simulink model "DroneSim"  (R2026a)
settings: Solver=ode45  StopTime=20
undefined symbols (not defined in the file): A, B, Cobs, Klqr, Kr, Lobs, pVec, T_eq, u_eq, windStr, x0
libraries: simulink x3, cstblocks_varying x3
settings Model: Creator=bryon  LastModifiedBy=bryon

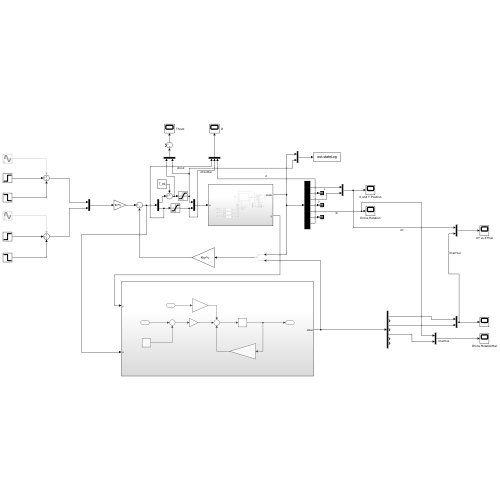
[thumbnail: Simulink's stored preview of the top-level diagram]
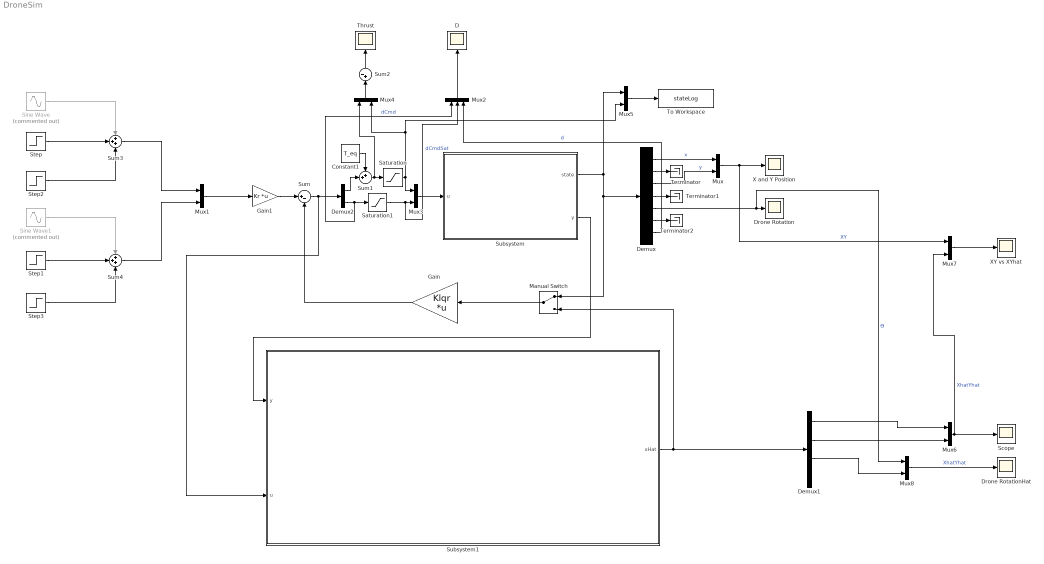
== system DroneSim ==
  Constant1 : Constant  Value=T_eq
  D : Scope
      settings: ActiveDisplayYMinimum=-0.1234265592827184  ActiveDisplayYMaximum=0.24991907295143939  DataLoggingVariableName=ScopeData6
  Demux : Demux  Outputs=7
  Demux1 : Demux  Outputs=7
  Demux2 : Demux  Outputs=2
  Drone Rotation : Scope
      settings: ActiveDisplayYMinimum=-1.627073692296509  ActiveDisplayYMaximum=1.6290895422795066  DataLoggingVariableName=ScopeData2
  Drone RotationHat : Scope
      settings: ActiveDisplayYMinimum=-3.0266243085418969  ActiveDisplayYMaximum=2.7501535670492685  DataLoggingVariableName=ScopeData10
  Gain : Gain  Gain=Klqr  Multiplication=Matrix(K*u)
  Gain1 : Gain  Gain=Kr  Multiplication=Matrix(K*u)
  Manual Switch : ManualSwitch
  Mux{,1,3..8} (8 alike) : Mux  Inputs=2
  Mux2 : Mux  Inputs=3
  Saturation : Saturate  UpperLimit=20  LowerLimit=0
  Saturation1 : Saturate  UpperLimit=.15  LowerLimit=-.15
  Scope : Scope
      settings: ActiveDisplayYMinimum=-1  ActiveDisplayYMaximum=1  DataLoggingVariableName=ScopeData4
  Sine Wave : Sin  Commented=on  Frequency=.5  SampleTime=0
  Sine Wave1 : Sin  Commented=on  Frequency=.5  Phase=pi/2  SampleTime=0
  Step : Step  Time=5  FinalValue=5  SampleTime=0
  Step1 : Step  Time=10  FinalValue=5  SampleTime=0
  Step2 : Step  Time=10  FinalValue=-5  SampleTime=0
  Step3 : Step  Time=15  FinalValue=-5  SampleTime=0
  Subsystem : Subsystem
  Subsystem1 : Subsystem
  Sum : Sum  Inputs=|+-
  Sum1 : Sum  Inputs=++|
  Sum2 : Sum  Inputs=-+|
  Sum3 : Sum  Inputs=+++
  Sum4 : Sum  Inputs=+++
  Terminator : Terminator
  Terminator1 : Terminator
  Terminator2 : Terminator
  Thrust : Scope
      settings: ActiveDisplayYMinimum=-3.5627589609078054  ActiveDisplayYMaximum=19.258872430937281  DataLoggingVariableName=ScopeData5
  To Workspace : ToWorkspace  VariableName=stateLog  SaveFormat=Timeseries  SampleTime=-1
  X and Y Position : Scope
      settings: ActiveDisplayYMinimum=-7.1769758544184414  ActiveDisplayYMaximum=11.233551342341229  DataLoggingVariableName=ScopeData3
  XY vs XYhat : Scope
      settings: ActiveDisplayYMinimum=-6.6188356438338474  ActiveDisplayYMaximum=6.5225549790711037  DataLoggingVariableName=ScopeData9
  wires:
  Demux/4 -> Terminator1/1
  Demux/6 -> Terminator2/1
  Demux/5 -> Mux8/1, Drone Rotation/1  "ϴ"
  Demux/2 -> Terminator/1
  Demux/3 -> Mux/2  "y"
  Demux/7 -> Mux2/3  "d"
  Mux/1 -> X and Y Position/1, Mux7/1  "XY"
  Demux/1 -> Mux/1  "x"
  Subsystem/1(state) -> Manual Switch/1, Demux/1, Mux5/1
  Gain/1 -> Sum/2
  Gain1/1 -> Sum/1
  Mux1/1 -> Gain1/1
  Mux2/1 -> D/1
  Constant1/1 -> Sum1/1
  Demux2/1 -> Sum1/2
  Sum1/1 -> Mux4/1, Saturation/1
  Saturation/1 -> Mux5/2, Mux4/2, Mux3/1
  Mux3/1 -> Subsystem/1(u)
  Demux2/2 -> Saturation1/1, Mux2/1  "dCmd"
  Saturation1/1 -> Mux2/2, Mux3/2  "dCmdSat"
  Sum2/1 -> Thrust/1
  Mux4/1 -> Sum2/2
  Mux5/1 -> To Workspace/1
  Step/1 -> Sum3/2
  Sum3/1 -> Mux1/1
  Step2/1 -> Sum3/3
  Step1/1 -> Sum4/2
  Sum4/1 -> Mux1/2
  Step3/1 -> Sum4/3
  Manual Switch/1 -> Gain/1
  Subsystem1/1(xHat) -> Demux1/1, Manual Switch/2
  Subsystem/2(y) -> Subsystem1/1(y)
  Demux1/1 -> Mux6/1
  Demux1/3 -> Mux6/2
  Mux6/1 -> Mux7/2, Scope/1  "XhatYhat"
  Mux7/1 -> XY vs XYhat/1
  Sum/1 -> Subsystem1/2(u), Demux2/1
  Mux8/1 -> Drone RotationHat/1  "XhatYhat"
  Demux1/5 -> Mux8/2
  Sine Wave/1 -> Sum3/1
  Sine Wave1/1 -> Sum4/1

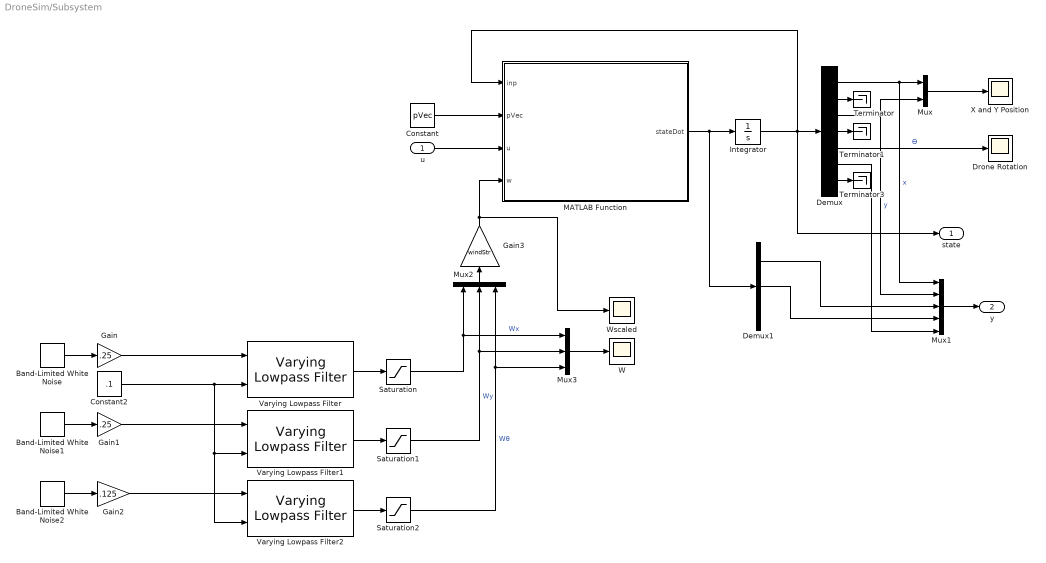
== system DroneSim/Subsystem ==
  u : Inport
  Band-Limited White Noise : simulink/Sources/Band-Limited White Noise  Cov=[0.1]  Ts=0.1  seed=[23341]
  Band-Limited White Noise1 : simulink/Sources/Band-Limited White Noise  Cov=[0.1]  Ts=0.1  seed=[47957]
  Band-Limited White Noise2 : simulink/Sources/Band-Limited White Noise  Cov=[0.1]  Ts=0.1  seed=[13468]
  Constant : Constant  Value=pVec
  Constant2 : Constant  Value=.1
  Demux : Demux  Outputs=7
  Demux1 : Demux  Outputs=7
  Drone Rotation : Scope
      settings: ActiveDisplayYMinimum=-13.749404737910847  ActiveDisplayYMaximum=123.74464264119766
  Gain : Gain  Gain=.25
  Gain1 : Gain  Gain=.25
  Gain2 : Gain  Gain=.125
  Gain3 : Gain  Gain=windStr
  Integrator : Integrator  InitialCondition=x0
  MATLAB Function : MATLAB Function  TreatAsAtomicUnit=on
  Mux : Mux  Inputs=2
  Mux1 : Mux  Inputs=5
  Mux2 : Mux  Inputs=3
  Mux3 : Mux  Inputs=3
  Saturation : Saturate
  Saturation1 : Saturate
  Saturation2 : Saturate
  Terminator : Terminator
  Terminator1 : Terminator
  Terminator3 : Terminator
  Varying Lowpass Filter : cstblocks_varying/Varying Lowpass Filter  N=1
      settings: LibrarySourceBlock=cstblocks/Linear Parameter Varying/Varying Lowpass Filter
  Varying Lowpass Filter1 : cstblocks_varying/Varying Lowpass Filter  N=1
      settings: LibrarySourceBlock=cstblocks/Linear Parameter Varying/Varying Lowpass Filter
  Varying Lowpass Filter2 : cstblocks_varying/Varying Lowpass Filter  N=1
      settings: LibrarySourceBlock=cstblocks/Linear Parameter Varying/Varying Lowpass Filter
  W : Scope
      settings: ActiveDisplayYMinimum=-1.2124820017506956  ActiveDisplayYMaximum=1.7686961340561902  DataLoggingVariableName=ScopeData7
  Wscaled : Scope
      settings: ActiveDisplayYMinimum=-1  ActiveDisplayYMaximum=1  DataLoggingVariableName=ScopeData8
  X and Y Position : Scope
      settings: ActiveDisplayYMinimum=-1  ActiveDisplayYMaximum=1
  state : Outport
  y : Outport  Port=2
  wires:
  Integrator/1 -> MATLAB Function/1(inp), state/1, Demux/1
  u/1 -> MATLAB Function/3(u)
  Mux/1 -> X and Y Position/1
  Constant/1 -> MATLAB Function/2(pVec)
  MATLAB Function/1(stateDot) -> Integrator/1, Demux1/1
  Demux/1 -> Mux1/1, Mux/1  "x"
  Demux/3 -> Mux1/2, Mux/2  "y"
  Demux/7 -> Terminator3/1
  Demux/5 -> Drone Rotation/1  "ϴ"
  Demux/6 -> Mux1/5
  Demux/2 -> Terminator/1
  Demux/4 -> Terminator1/1
  Mux2/1 -> Gain3/1
  Band-Limited White Noise/1 -> Gain/1
  Gain/1 -> Varying Lowpass Filter/1
  Constant2/1 -> Varying Lowpass Filter2/2, Varying Lowpass Filter1/2, Varying Lowpass Filter/2
  Varying Lowpass Filter/1 -> Saturation/1
  Saturation/1 -> Mux3/1, Mux2/1  "Wx"
  Gain1/1 -> Varying Lowpass Filter1/1
  Saturation1/1 -> Mux3/2, Mux2/2  "Wy"
  Band-Limited White Noise1/1 -> Gain1/1
  Varying Lowpass Filter1/1 -> Saturation1/1
  Mux3/1 -> W/1
  Varying Lowpass Filter2/1 -> Saturation2/1
  Gain2/1 -> Varying Lowpass Filter2/1
  Band-Limited White Noise2/1 -> Gain2/1
  Saturation2/1 -> Mux2/3, Mux3/3  "Wθ"
  Gain3/1 -> Wscaled/1, MATLAB Function/4(w)
  Mux1/1 -> y/1
  Demux1/2 -> Mux1/3
  Demux1/4 -> Mux1/4

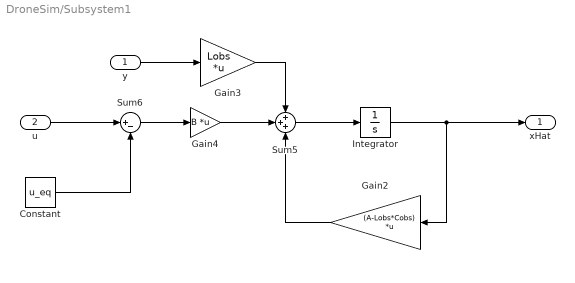
== system DroneSim/Subsystem1 ==
  y : Inport
  u : Inport  Port=2
  Constant : Constant  Value=u_eq
  Gain2 : Gain  Gain=(A-Lobs*Cobs)  Multiplication=Matrix(K*u)
  Gain3 : Gain  Gain=Lobs  Multiplication=Matrix(K*u)
  Gain4 : Gain  Gain=B  Multiplication=Matrix(K*u)
  Integrator : Integrator
  Sum5 : Sum  Inputs=+++
  Sum6 : Sum  Inputs=|+-
  xHat : Outport
  wires:
  Gain2/1 -> Sum5/3
  Integrator/1 -> xHat/1, Gain2/1
  Sum5/1 -> Integrator/1
  Gain4/1 -> Sum5/2
  Gain3/1 -> Sum5/1
  y/1 -> Gain3/1
  Constant/1 -> Sum6/2
  u/1 -> Sum6/1
  Sum6/1 -> Gain4/1

== matlab function DroneSim/Subsystem/MATLAB Function ==
  data: inp input; pVec input; u input; stateDot output; w input
function stateDot = rhsDrone(inp, pVec, u, w)

stateDot = zeros(7,1);

% State variables
x_dot 		= inp(2);
y_dot 		= inp(4);
theta 		= inp(5);
theta_dot 	= inp(6);
d 			= inp(7);

% System Parameters
mc 	        = pVec(1);
g 	        = pVec(2);
IG 	        = pVec(3);
tauRack     = pVec(4);

% Inputs
T           = u(1);
dcmd        = u(2);

M = [
	mc 0 0;
	0 mc 0;
	0 0 IG;
	];
	
Fx_wind  = w(1);
Fy_wind  = w(2);
Tau_wind = w(3);

R = [
    -T*sin(theta) + Fx_wind;
     T*cos(theta) - mc*g + Fy_wind;
     T*d + Tau_wind
];

ddot = M\R;

stateDot(1) = x_dot;
stateDot(2) = ddot(1);
stateDot(3) = y_dot;
stateDot(4) = ddot(2);
stateDot(5) = theta_dot;
stateDot(6) = ddot(3);
stateDot(7) = (dcmd - d)/tauRack;

end
